simulink model "CL_Xpro_model"  (Simulink 9.1)
settings: Solver=ode45  StartTime=0.0  StopTime=total_time  RelTol=1e-3  EnableMultiTasking=on
values from neighbouring files (symbols this model uses):
  a1 = 16.235    [LoadQuadrotorConst_XPro1a.m]
  a2 = 17.912    [LoadQuadrotorConst_XPro1a.m]
  a3 = 17.914    [LoadQuadrotorConst_XPro1a.m]
  a4 = 18.161    [LoadQuadrotorConst_XPro1a.m]
  b1 = -0.5036    [LoadQuadrotorConst_XPro1a.m]
  b2 = -12.728    [LoadQuadrotorConst_XPro1a.m]
  b3 = -6.5646    [LoadQuadrotorConst_XPro1a.m]
  b4 = -7.4637    [LoadQuadrotorConst_XPro1a.m]
  c = 0.0002    [LoadQuadrotorConst_XPro1a.m]
  c_mi_x = 170*0    (= 0)    [LoadQuadrotorConst_XPro1a.m]
  c_mi_y = 170*0    (= 0)    [LoadQuadrotorConst_XPro1a.m]
  c_mi_z = 40*0    (= 0)    [LoadQuadrotorConst_XPro1a.m]
  co_x = 1.7*0    (= 0)    [LoadQuadrotorConst_XPro1a.m]
  co_y = 1.7*0    (= 0)    [LoadQuadrotorConst_XPro1a.m]
  co_z = 90.7*0    (= 0)    [LoadQuadrotorConst_XPro1a.m]
  controller = 0    [main_sim.m]
  d = 0.5    [LoadQuadrotorConst_XPro1a.m]
  d_omega_R10 = 9.1275    [initial_conditions.m]
  d_omega_R20 = 8.955    [initial_conditions.m]
  d_omega_R30 = 8.61    [initial_conditions.m]
  d_omega_R40 = 8.543    [initial_conditions.m]
  dfi_0 = -0    (= 0)    [initial_conditions.m]
  dpsi_0 = 0    [initial_conditions.m]
  dtheta_0 = 0    [initial_conditions.m]
  dx_0 = 0    [initial_conditions.m]
  dy_0 = 0    [initial_conditions.m]
  dz_0 = 0    [initial_conditions.m]
  f = 5e-6    (= 5e-06)    [LoadQuadrotorConst_XPro1a.m]
  factor = 0.35    [main_sim.m]
  fi_0 = 0    [initial_conditions.m]
  g = 9.807    [K.mat]    (also in LoadQuadrotorConst_XPro1a.m = 0.0008)
  ga = g    [LoadQuadrotorConst_XPro1a.m]
  Gamma = usample(gamma)    [LoadQuadrotorConst_XPro1a.m]
  h = -0.0282    [LoadQuadrotorConst_XPro1a.m]
  input_disturbance = [2 0.4 0.4 0.05]    [K.mat]
  invJac = inv(Jac)    [LoadQuadrotorConst_XPro1a.m]
  Ixx = usample(Ix)    [LoadQuadrotorConst_XPro1a.m]
  Iyy = usample(Iy)    [LoadQuadrotorConst_XPro1a.m]
  Izz = usample(Iz)    [LoadQuadrotorConst_XPro1a.m]
  Jr = 4.86851*0.1    (= 0.486851)    [LoadQuadrotorConst_XPro1a.m]
  L = usample(lx)    [LoadQuadrotorConst_XPro1a.m]
  m = m_nom    [LoadQuadrotorConst_XPro1a.m]
  psi_0 = 0    [initial_conditions.m]
  sensor_noise_weights = [0.1 0.1 0.1 0.01 0.01 0.01 0.0873 0.0873 0.0873 0.00873 0.00873 0.00873]    [K.mat]
  Tau = usample(tau)    [LoadQuadrotorConst_XPro1a.m]
  theta_0 = 0    [initial_conditions.m]
  u_op = [20.5947 0 0 0]    [K.mat]
  V1_WP = 9.1275    [initial_conditions.m]
  V2_WP = 8.955    [initial_conditions.m]
  V3_WP = 8.61    [initial_conditions.m]
  V4_WP = 8.543    [initial_conditions.m]
  x_0 = 0    [initial_conditions.m]
  x_des = [1; 1; 1; 0; 0; 0; 0; 0; pi/12; 0; 0; 0]    [main_sim.m]
  y_0 = 0    [initial_conditions.m]
  z_0 = 0    [initial_conditions.m]
undefined symbols (not defined in the file or in its folder): k, K_lqr
settings Model: SuppressorTable=22 serialization::archive 11 0 6 0 0 0 0 0  Creator=Jake  LastModifiedBy=michaelwang
settings DataIOCC: LimitDataPoints=on  SignalLoggingSaveFormat=ModelDataLogs
settings OptimizationCC: InitFltsAndDblsToZero=on
settings DebuggingCC: SaveWithParameterizedLinksMsg=none  SignalResolutionControl=TryResolveAllWithWarning  SolverPrmCheckMsg=warning  MultiTaskDSMMsg=warning  MultiTaskCondExecSysMsg=none  FcnCallInpInsideContextMsg=warning
settings SFSimCC: SimParseCustomCode=off
settings GRTTargetCC: TargetFcnLib=ansi_tfl_tmw.mat

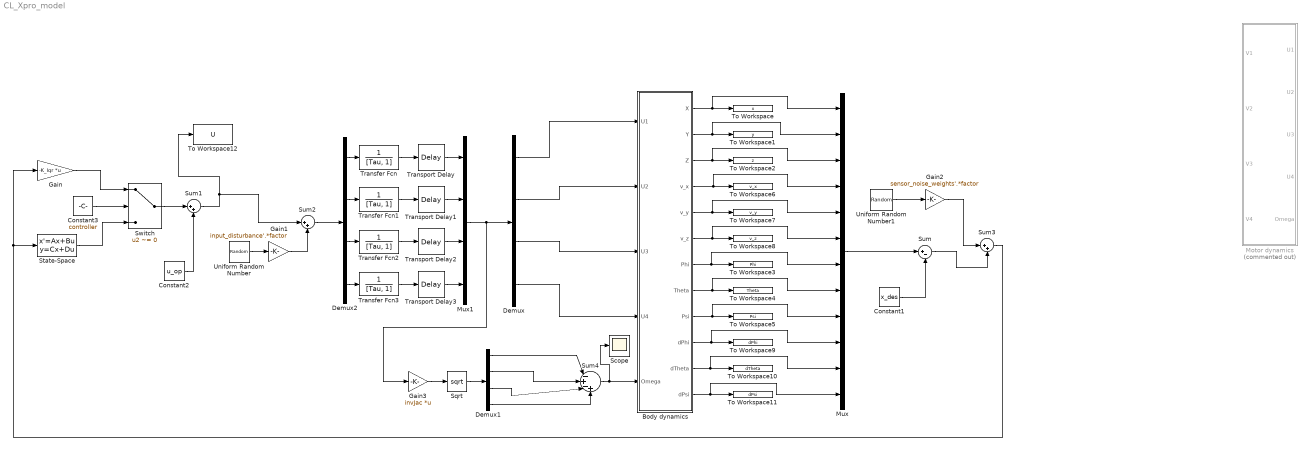
== system CL_Xpro_model ==
  Body dynamics : Subsystem
  Constant1 : Constant  Value=x_des
  Constant2 : Constant  Value=u_op
  Constant3 : Constant  Value=controller
  Demux : Demux
  Demux1 : Demux
  Demux2 : Demux
  Gain : Gain  Gain=-K_lqr  Multiplication=Matrix(K*u)
  Gain1 : Gain  Gain=input_disturbance'.*factor
  Gain2 : Gain  Gain=sensor_noise_weights'.*factor
  Gain3 : Gain  Gain=invJac  Multiplication=Matrix(K*u)
  Motor dynamics : Subsystem  Commented=on
  Mux : Mux  Inputs=12
  Mux1 : Mux
  Scope : Scope
  Sqrt : Sqrt  SaturateOnIntegerOverflow=on
  State-Space : StateSpace  A=k.A  B=k.B  C=k.C  D=k.D  InitialCondition=0
  Sum : Sum  Inputs=|+-
  Sum1 : Sum  Inputs=|++
  Sum2 : Sum  Inputs=|++
  Sum3 : Sum  Inputs=|++
  Sum4 : Sum  Inputs=|-+-+
  Switch : Switch  Criteria=u2 ~= 0
  To Workspace : ToWorkspace  VariableName=x  SaveFormat=Timeseries  SampleTime=-1
  To Workspace1 : ToWorkspace  VariableName=y  SaveFormat=Timeseries  SampleTime=-1
  To Workspace10 : ToWorkspace  VariableName=dTheta  SaveFormat=Timeseries  SampleTime=-1
  To Workspace11 : ToWorkspace  VariableName=dPsi  SaveFormat=Timeseries  SampleTime=-1
  To Workspace12 : ToWorkspace  VariableName=U  SaveFormat=Timeseries  SampleTime=-1
  To Workspace2 : ToWorkspace  VariableName=z  SaveFormat=Timeseries  SampleTime=-1
  To Workspace3 : ToWorkspace  VariableName=Phi  SaveFormat=Timeseries  SampleTime=-1
  To Workspace4 : ToWorkspace  VariableName=Theta  SaveFormat=Timeseries  SampleTime=-1
  To Workspace5 : ToWorkspace  VariableName=Psi  SaveFormat=Timeseries  SampleTime=-1
  To Workspace6 : ToWorkspace  VariableName=v_x  SaveFormat=Timeseries  SampleTime=-1
  To Workspace7 : ToWorkspace  VariableName=v_y  SaveFormat=Timeseries  SampleTime=-1
  To Workspace8 : ToWorkspace  VariableName=v_z  SaveFormat=Timeseries  SampleTime=-1
  To Workspace9 : ToWorkspace  VariableName=dPhi  SaveFormat=Timeseries  SampleTime=-1
  Transfer Fcn{,1..3} (4 alike) : TransferFcn  Denominator=[Tau, 1]
  Transport Delay{,1..3} (4 alike) : TransportDelay  DelayTime=Gamma
  Uniform Random Number : UniformRandomNumber  Minimum=ones(length(input_disturbance),1).*-1  Maximum=ones(length(input_disturbance), 1)  Seed=abs(round(rand().*10))  SampleTime=0.1
  Uniform Random Number1 : UniformRandomNumber  Minimum=ones(length(sensor_noise_weights),1).*-1  Maximum=ones(length(sensor_noise_weights), 1)  Seed=abs(round(rand().*10))  SampleTime=0.1
  wires:
  Body dynamics/1(X) -> Mux/1, To Workspace/1
  Body dynamics/3(Z) -> Mux/3, To Workspace2/1
  Body dynamics/2(Y) -> Mux/2, To Workspace1/1
  Demux/1 -> Body dynamics/1(U1)
  Demux/2 -> Body dynamics/2(U2)
  Demux/3 -> Body dynamics/3(U3)
  Demux/4 -> Body dynamics/4(U4)
  Body dynamics/12(dPsi) -> Mux/12, To Workspace11/1
  Body dynamics/11(dTheta) -> Mux/11, To Workspace10/1
  Body dynamics/10(dPhi) -> Mux/10, To Workspace9/1
  Body dynamics/7(Phi) -> Mux/7, To Workspace3/1
  Body dynamics/8(Theta) -> Mux/8, To Workspace4/1
  Body dynamics/9(Psi) -> Mux/9, To Workspace5/1
  Body dynamics/4(v_x) -> Mux/4, To Workspace6/1
  Body dynamics/5(v_y) -> Mux/5, To Workspace7/1
  Body dynamics/6(v_z) -> Mux/6, To Workspace8/1
  Mux/1 -> Sum/1
  Constant1/1 -> Sum/2
  Sum1/1 -> Sum2/1, To Workspace12/1
  Constant2/1 -> Sum1/2
  Constant3/1 -> Switch/2
  Switch/1 -> Sum1/1
  State-Space/1 -> Switch/3
  Gain/1 -> Switch/1
  Uniform Random Number/1 -> Gain1/1
  Gain1/1 -> Sum2/2
  Uniform Random Number1/1 -> Gain2/1
  Gain2/1 -> Sum3/1
  Sum3/1 -> State-Space/1, Gain/1
  Sum/1 -> Sum3/2
  Gain3/1 -> Sqrt/1
  Sqrt/1 -> Demux1/1
  Sum4/1 -> Scope/1, Body dynamics/5(Omega)
  Demux1/1 -> Sum4/1
  Demux1/2 -> Sum4/2
  Demux1/4 -> Sum4/4
  Demux1/3 -> Sum4/3
  Transfer Fcn/1 -> Transport Delay/1
  Sum2/1 -> Demux2/1
  Demux2/1 -> Transfer Fcn/1
  Transfer Fcn1/1 -> Transport Delay1/1
  Transfer Fcn2/1 -> Transport Delay2/1
  Transfer Fcn3/1 -> Transport Delay3/1
  Demux2/4 -> Transfer Fcn3/1
  Demux2/3 -> Transfer Fcn2/1
  Demux2/2 -> Transfer Fcn1/1
  Transport Delay/1 -> Mux1/1
  Transport Delay1/1 -> Mux1/2
  Transport Delay2/1 -> Mux1/3
  Transport Delay3/1 -> Mux1/4
  Mux1/1 -> Gain3/1, Demux/1

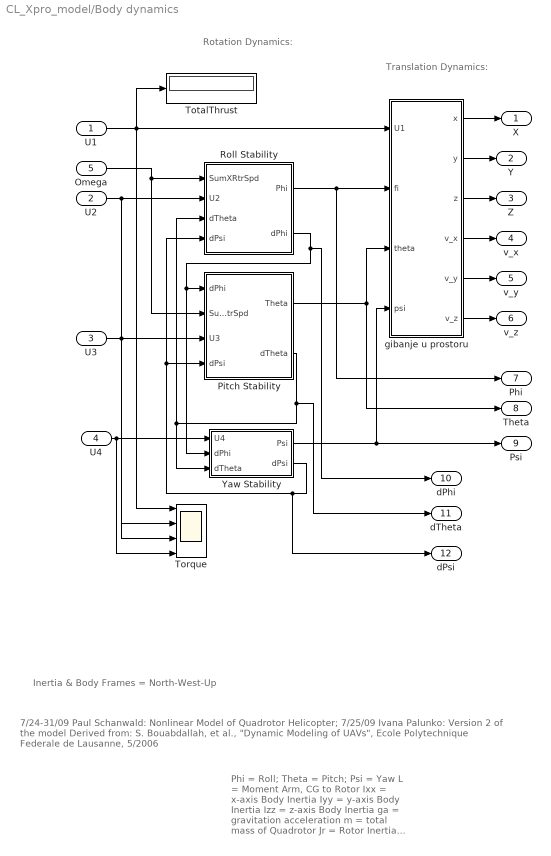
== system CL_Xpro_model/Body dynamics ==
  note: Inertia & Body Frames = North-West-Up
  note: Rotation
      | Dynamics:
  note: Translation
      | Dynamics:
  note: Phi = Roll; Theta = Pitch; Psi = Yaw
      | L = Moment Arm, CG to Rotor
      | Ixx = x-axis Body Inertia
      | Iyy = y-axis Body Inertia
      | Izz = z-axis Body Inertia
      | ga = gravitation acceleration
      | m = total mass of Quadrotor
      | Jr = Rotor Inertia
      | a,b = Volts-to-Rotor Speed Consts
      | c,d,e = RtrSpd-to-Thrust Fcn Consts
      | f,g,h = RtrSpd-to-Drag Fcn Consts
      | Tau = Motor Time Const
  note: 7/24-31/09  Paul Schanwald:  Nonlinear Model of Quadrotor Helicopter; 7/25/09 Ivana Palunko: Version 2 of the model
      | Derived from: S. Bouabdallah, et al., "Dynamic Modeling of UAVs", Ecole Polytechnique Federale de Lausanne, 5/2006
  U1 : Inport
  U2 : Inport  Port=2
  U3 : Inport  Port=3
  U4 : Inport  Port=4
  Omega : Inport  Port=5
  Pitch Stability : Subsystem
  Roll Stability : Subsystem
  Torque : Scope  NumInputPorts=4
  TotalThrust : Display
  Yaw Stability : Subsystem
  gibanje u prostoru : Subsystem
  X : Outport
  Y : Outport  Port=2
  Z : Outport  Port=3
  v_x : Outport  Port=4
  v_y : Outport  Port=5
  v_z : Outport  Port=6
  Phi : Outport  Port=7
  Theta : Outport  Port=8
  Psi : Outport  Port=9
  dPhi : Outport  Port=10
  dTheta : Outport  Port=11
  dPsi : Outport  Port=12
  wires:
  U4/1 -> Yaw Stability/1(U4), Torque/4
  U3/1 -> Pitch Stability/3(U3), Torque/3
  U1/1 -> TotalThrust/1, gibanje u prostoru/1(U1), Torque/1
  gibanje u prostoru/3(z) -> Z/1
  gibanje u prostoru/2(y) -> Y/1
  gibanje u prostoru/1(x) -> X/1
  U2/1 -> Roll Stability/2(U2), Torque/2
  Omega/1 -> Roll Stability/1(SumXRtrSpd), Pitch Stability/2(SumYRtrSpd)
  Roll Stability/2(dPhi) -> dPhi/1, Pitch Stability/1(dPhi), Yaw Stability/2(dPhi)
  Pitch Stability/2(dTheta) -> dTheta/1, Yaw Stability/3(dTheta), Roll Stability/3(dTheta)
  Yaw Stability/2(dPsi) -> dPsi/1, Roll Stability/4(dPsi), Pitch Stability/4(dPsi)
  Roll Stability/1(Phi) -> gibanje u prostoru/2(fi), Phi/1
  Pitch Stability/1(Theta) -> gibanje u prostoru/3(theta), Theta/1
  Yaw Stability/1(Psi) -> Psi/1, gibanje u prostoru/4(psi)
  gibanje u prostoru/6(v_z) -> v_z/1
  gibanje u prostoru/4(v_x) -> v_x/1
  gibanje u prostoru/5(v_y) -> v_y/1

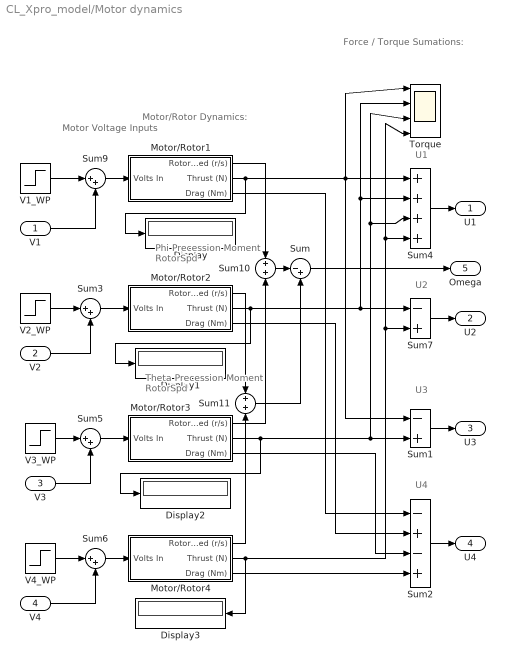
== system CL_Xpro_model/Motor dynamics ==
  note: Theta Precession
      | Moment RotorSpd
  note: Phi Precession
      | Moment RotorSpd
  note: Motor/Rotor
      | Dynamics:
  note: Force / Torque
      | Sumations:
  note: Motor
      | Voltage
      | Inputs
  note: U4
  note: U3
  note: U2
  note: U1
  V1 : Inport
  V2 : Inport  Port=2
  V3 : Inport  Port=3
  V4 : Inport  Port=4
  Display{,1..3} (4 alike) : Display
  Motor/Rotor1 : Subsystem
  Motor/Rotor2 : Subsystem
  Motor/Rotor3 : Subsystem
  Motor/Rotor4 : Subsystem
  Sum : Sum  Inputs=|-+
  Sum1 : Sum  Inputs=-+
  Sum10 : Sum  Inputs=+|+
  Sum11 : Sum  Inputs=+|+
  Sum2 : Sum  Inputs=-+-+
  Sum{3,5..6,9} (4 alike) : Sum  Inputs=|++
  Sum4 : Sum  Inputs=++++
  Sum7 : Sum  Inputs=-+
  Torque : Scope  NumInputPorts=4
  V1_WP : Step  Time=0  Before=V1_WP  After=V1_WP  SampleTime=0
  V2_WP : Step  Time=0  Before=V2_WP  After=V2_WP  SampleTime=0
  V3_WP : Step  Time=0  Before=V3_WP  After=V3_WP  SampleTime=0
  V4_WP : Step  Time=0  Before=V4_WP  After=V4_WP  SampleTime=0
  U1 : Outport
  U2 : Outport  Port=2
  U3 : Outport  Port=3
  U4 : Outport  Port=4
  Omega : Outport  Port=5
  wires:
  Sum11/1 -> Sum/2
  Sum10/1 -> Sum/1
  Motor/Rotor4/1(Rotor Speed (r/s)) -> Sum11/2
  Motor/Rotor4/2(Thrust (N)) -> Display3/1, Torque/4, Sum4/4, Sum7/2
  Motor/Rotor4/3(Drag (Nm)) -> Sum2/4
  Motor/Rotor3/3(Drag (Nm)) -> Sum2/3
  Motor/Rotor3/1(Rotor Speed (r/s)) -> Sum10/2
  Motor/Rotor3/2(Thrust (N)) -> Display2/1, Torque/3, Sum4/3, Sum1/2
  Motor/Rotor2/1(Rotor Speed (r/s)) -> Sum11/1
  Motor/Rotor2/3(Drag (Nm)) -> Sum2/2
  Motor/Rotor2/2(Thrust (N)) -> Display1/1, Torque/2, Sum4/2, Sum7/1
  Motor/Rotor1/1(Rotor Speed (r/s)) -> Sum10/1
  Motor/Rotor1/3(Drag (Nm)) -> Sum2/1
  Motor/Rotor1/2(Thrust (N)) -> Display/1, Sum4/1, Torque/1, Sum1/1
  Sum4/1 -> U1/1
  Sum/1 -> Omega/1
  Sum7/1 -> U2/1
  Sum1/1 -> U3/1
  Sum2/1 -> U4/1
  Sum9/1 -> Motor/Rotor1/1(Volts In)
  V1_WP/1 -> Sum9/1
  V2_WP/1 -> Sum3/1
  Sum3/1 -> Motor/Rotor2/1(Volts In)
  V3_WP/1 -> Sum5/1
  Sum5/1 -> Motor/Rotor3/1(Volts In)
  V4_WP/1 -> Sum6/1
  Sum6/1 -> Motor/Rotor4/1(Volts In)
  V1/1 -> Sum9/2
  V2/1 -> Sum3/2
  V3/1 -> Sum5/2
  V4/1 -> Sum6/2

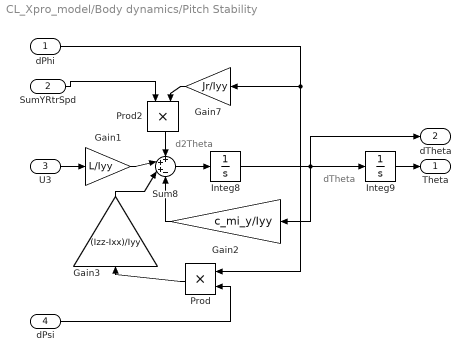
== system CL_Xpro_model/Body dynamics/Pitch Stability ==
  note: d2Theta
  note: dTheta
  dPhi : Inport
  SumYRtrSpd : Inport  Port=2
  U3 : Inport  Port=3
  dPsi : Inport  Port=4
  Gain1 : Gain  Gain=L/Iyy
  Gain2 : Gain  Gain=c_mi_y/Iyy
  Gain3 : Gain  Gain=(Izz-Ixx)/Iyy
  Gain7 : Gain  Gain=Jr/Iyy
  Integ8 : Integrator  InitialCondition=dtheta_0
  Integ9 : Integrator  InitialCondition=theta_0  UpperSaturationLimit=pi/2  LowerSaturationLimit=-pi/2
  Prod : Product  RndMeth=Zero
  Prod2 : Product  RndMeth=Zero
  Sum8 : Sum  Inputs=+++-
  Theta : Outport
  dTheta : Outport  Port=2
  wires:
  Gain2/1 -> Sum8/4
  dPhi/1 -> Prod/1, Gain7/1
  Integ9/1 -> Theta/1
  U3/1 -> Gain1/1
  SumYRtrSpd/1 -> Prod2/1
  dPsi/1 -> Prod/2
  Integ8/1 -> dTheta/1, Integ9/1, Gain2/1
  Sum8/1 -> Integ8/1
  Gain1/1 -> Sum8/2
  Gain7/1 -> Prod2/2
  Gain3/1 -> Sum8/3
  Prod/1 -> Gain3/1
  Prod2/1 -> Sum8/1

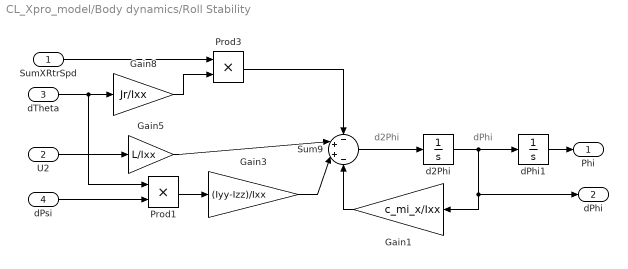
== system CL_Xpro_model/Body dynamics/Roll Stability ==
  note: d2Phi
  note: dPhi
  SumXRtrSpd : Inport
  U2 : Inport  Port=2
  dTheta : Inport  Port=3
  dPsi : Inport  Port=4
  Gain1 : Gain  Gain=c_mi_x/Ixx
  Gain3 : Gain  Gain=(Iyy-Izz)/Ixx
  Gain5 : Gain  Gain=L/Ixx
  Gain8 : Gain  Gain=Jr/Ixx
  Prod1 : Product  RndMeth=Zero
  Prod3 : Product  RndMeth=Zero
  Sum9 : Sum  Inputs=-++-
  d2Phi : Integrator  InitialCondition=dfi_0
  dPhi1 : Integrator  InitialCondition=fi_0  UpperSaturationLimit=pi/2  LowerSaturationLimit=-pi/2
  Phi : Outport
  dPhi : Outport  Port=2
  wires:
  dPsi/1 -> Prod1/2
  dTheta/1 -> Prod1/1, Gain8/1
  Prod3/1 -> Sum9/1
  SumXRtrSpd/1 -> Prod3/1
  Gain8/1 -> Prod3/2
  dPhi1/1 -> Phi/1
  U2/1 -> Gain5/1
  d2Phi/1 -> Gain1/1, dPhi/1, dPhi1/1
  Sum9/1 -> d2Phi/1
  Gain5/1 -> Sum9/2
  Gain1/1 -> Sum9/4
  Gain3/1 -> Sum9/3
  Prod1/1 -> Gain3/1

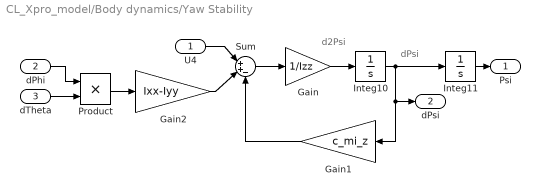
== system CL_Xpro_model/Body dynamics/Yaw Stability ==
  note: dPsi
  note: d2Psi
  U4 : Inport
  dPhi : Inport  Port=2
  dTheta : Inport  Port=3
  Gain : Gain  Gain=1/Izz
  Gain1 : Gain  Gain=c_mi_z
  Gain2 : Gain  Gain=Ixx-Iyy
  Integ10 : Integrator  InitialCondition=dpsi_0
  Integ11 : Integrator  InitialCondition=psi_0
  Product : Product  RndMeth=Zero
  Sum : Sum  Inputs=|++-
  Psi : Outport
  dPsi : Outport  Port=2
  wires:
  Sum/1 -> Gain/1
  U4/1 -> Sum/1
  Integ11/1 -> Psi/1
  Gain/1 -> Integ10/1
  Integ10/1 -> Gain1/1, dPsi/1, Integ11/1
  Gain1/1 -> Sum/3
  Gain2/1 -> Sum/2
  dPhi/1 -> Product/1
  dTheta/1 -> Product/2
  Product/1 -> Gain2/1

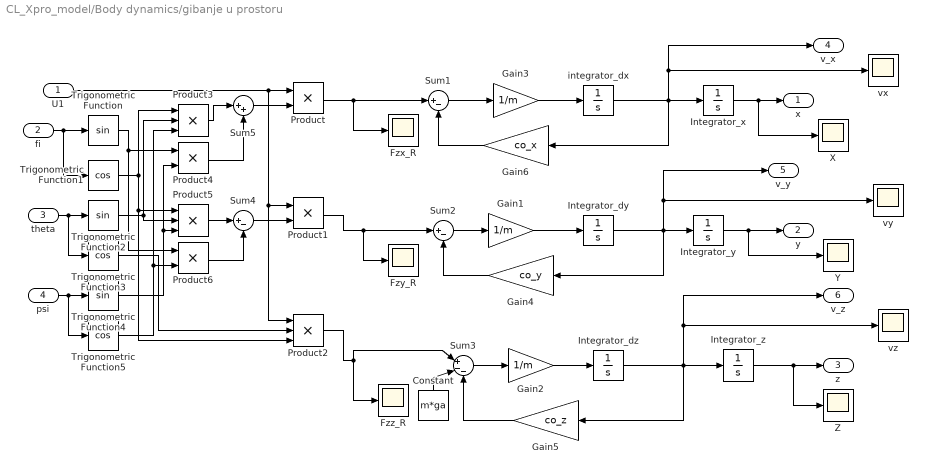
== system CL_Xpro_model/Body dynamics/gibanje u prostoru ==
  U1 : Inport
  fi : Inport  Port=2
  theta : Inport  Port=3
  psi : Inport  Port=4
  Constant : Constant  Value=m*ga
  Fzx_R : Scope
  Fzy_R : Scope
  Fzz_R : Scope
  Gain1 : Gain  Gain=1/m
  Gain2 : Gain  Gain=1/m
  Gain3 : Gain  Gain=1/m
  Gain4 : Gain  Gain=co_y
  Gain5 : Gain  Gain=co_z
  Gain6 : Gain  Gain=co_x
  Integrator_dy : Integrator  InitialCondition=dy_0  LimitOutput=on  UpperSaturationLimit=10  LowerSaturationLimit=-10
  Integrator_dz : Integrator  InitialCondition=dz_0  LimitOutput=on  UpperSaturationLimit=10  LowerSaturationLimit=-10
  Integrator_x : Integrator  InitialCondition=x_0
  Integrator_y : Integrator  InitialCondition=y_0
  Integrator_z : Integrator  InitialCondition=z_0
  Product{,1,4,6} (4 alike) : Product  RndMeth=Zero
  Product2 : Product  Inputs=3  RndMeth=Zero
  Product3 : Product  Inputs=3  RndMeth=Zero
  Product5 : Product  Inputs=3  RndMeth=Zero
  Sum1 : Sum  Inputs=|+-
  Sum2 : Sum  Inputs=|+-
  Sum3 : Sum  Inputs=|+--
  Sum4 : Sum  Inputs=|+-
  Sum5 : Sum  Inputs=|++
  Trigonometric Function : Trigonometry
  Trigonometric Function1 : Trigonometry  Operator=cos
  Trigonometric Function2 : Trigonometry
  Trigonometric Function3 : Trigonometry  Operator=cos
  Trigonometric Function4 : Trigonometry
  Trigonometric Function5 : Trigonometry  Operator=cos
  X : Scope
  Y : Scope
  Z : Scope
  integrator_dx : Integrator  InitialCondition=dx_0  LimitOutput=on  UpperSaturationLimit=10  LowerSaturationLimit=-10
  vx : Scope
  vy : Scope
  vz : Scope
  x : Outport
  y : Outport  Port=2
  z : Outport  Port=3
  v_x : Outport  Port=4
  v_y : Outport  Port=5
  v_z : Outport  Port=6
  wires:
  Gain5/1 -> Sum3/3
  Constant/1 -> Sum3/2
  Gain4/1 -> Sum2/2
  Sum3/1 -> Gain2/1
  Gain6/1 -> Sum1/2
  Product2/1 -> Sum3/1, Fzz_R/1
  Sum2/1 -> Gain1/1
  Product1/1 -> Fzy_R/1, Sum2/1
  Gain2/1 -> Integrator_dz/1
  Sum1/1 -> Gain3/1
  Product/1 -> Fzx_R/1, Sum1/1
  U1/1 -> Product/1, Product1/1, Product2/1
  Integrator_y/1 -> Y/1, y/1
  Integrator_x/1 -> X/1, x/1
  Integrator_z/1 -> Z/1, z/1
  integrator_dx/1 -> Gain6/1, vx/1, v_x/1, Integrator_x/1
  Integrator_dy/1 -> Gain4/1, Integrator_y/1, vy/1, v_y/1
  Integrator_dz/1 -> vz/1, v_z/1, Gain5/1, Integrator_z/1
  Gain1/1 -> Integrator_dy/1
  Gain3/1 -> integrator_dx/1
  Sum4/1 -> Product1/2
  Sum5/1 -> Product/2
  Product3/1 -> Sum5/1
  Product4/1 -> Sum5/2
  Product5/1 -> Sum4/1
  Product6/1 -> Sum4/2
  psi/1 -> Trigonometric Function4/1, Trigonometric Function5/1
  theta/1 -> Trigonometric Function2/1, Trigonometric Function3/1
  fi/1 -> Trigonometric Function/1, Trigonometric Function1/1
  Trigonometric Function/1 -> Product4/1, Product6/1
  Trigonometric Function1/1 -> Product3/1, Product5/1, Product2/3
  Trigonometric Function2/1 -> Product3/2, Product5/2
  Trigonometric Function5/1 -> Product3/3, Product6/2
  Trigonometric Function4/1 -> Product4/2, Product5/3
  Trigonometric Function3/1 -> Product2/2

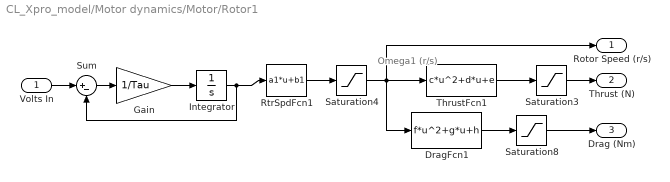
== system CL_Xpro_model/Motor dynamics/Motor/Rotor1 ==
  note: Omega1
      | (r/s)
  Volts In : Inport
  DragFcn1 : Fcn  Expr=f*u^2+g*u+h
  Gain : Gain  Gain=1/Tau
  Integrator : Integrator  InitialCondition=d_omega_R10
  RtrSpdFcn1 : Fcn  Expr=a1*u+b1
  Saturation3 : Saturate  UpperLimit=15  LowerLimit=0
  Saturation4 : Saturate  UpperLimit=250  LowerLimit=0
  Saturation8 : Saturate  UpperLimit=1  LowerLimit=0
  Sum : Sum  Inputs=|+-
  ThrustFcn1 : Fcn  Expr=c*u^2+d*u+e
  Rotor Speed (r/s) : Outport
  Thrust (N) : Outport  Port=2
  Drag (Nm) : Outport  Port=3
  wires:
  Volts In/1 -> Sum/1
  Sum/1 -> Gain/1
  Integrator/1 -> RtrSpdFcn1/1, Sum/2
  Gain/1 -> Integrator/1
  Saturation3/1 -> Thrust (N)/1
  Saturation8/1 -> Drag (Nm)/1
  DragFcn1/1 -> Saturation8/1
  Saturation4/1 -> Rotor Speed (r/s)/1, DragFcn1/1, ThrustFcn1/1
  RtrSpdFcn1/1 -> Saturation4/1
  ThrustFcn1/1 -> Saturation3/1

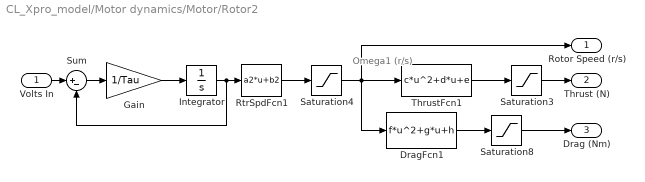
== system CL_Xpro_model/Motor dynamics/Motor/Rotor2 ==
  note: Omega1
      | (r/s)
  Volts In : Inport
  DragFcn1 : Fcn  Expr=f*u^2+g*u+h
  Gain : Gain  Gain=1/Tau
  Integrator : Integrator  InitialCondition=d_omega_R20
  RtrSpdFcn1 : Fcn  Expr=a2*u+b2
  Saturation3 : Saturate  UpperLimit=15  LowerLimit=0
  Saturation4 : Saturate  UpperLimit=250  LowerLimit=0
  Saturation8 : Saturate  UpperLimit=1  LowerLimit=0
  Sum : Sum  Inputs=|+-
  ThrustFcn1 : Fcn  Expr=c*u^2+d*u+e
  Rotor Speed (r/s) : Outport
  Thrust (N) : Outport  Port=2
  Drag (Nm) : Outport  Port=3
  wires:
  Volts In/1 -> Sum/1
  Sum/1 -> Gain/1
  Integrator/1 -> RtrSpdFcn1/1, Sum/2
  Gain/1 -> Integrator/1
  Saturation3/1 -> Thrust (N)/1
  Saturation8/1 -> Drag (Nm)/1
  DragFcn1/1 -> Saturation8/1
  ThrustFcn1/1 -> Saturation3/1
  Saturation4/1 -> Rotor Speed (r/s)/1, DragFcn1/1, ThrustFcn1/1
  RtrSpdFcn1/1 -> Saturation4/1

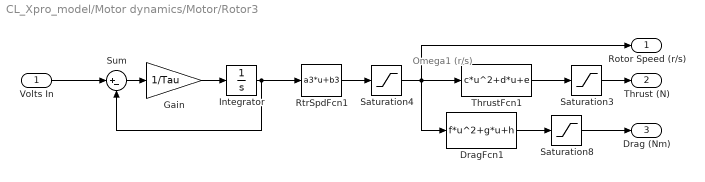
== system CL_Xpro_model/Motor dynamics/Motor/Rotor3 ==
  note: Omega1
      | (r/s)
  Volts In : Inport
  DragFcn1 : Fcn  Expr=f*u^2+g*u+h
  Gain : Gain  Gain=1/Tau
  Integrator : Integrator  InitialCondition=d_omega_R30
  RtrSpdFcn1 : Fcn  Expr=a3*u+b3
  Saturation3 : Saturate  UpperLimit=15  LowerLimit=0
  Saturation4 : Saturate  UpperLimit=250  LowerLimit=0
  Saturation8 : Saturate  UpperLimit=1  LowerLimit=0
  Sum : Sum  Inputs=|+-
  ThrustFcn1 : Fcn  Expr=c*u^2+d*u+e
  Rotor Speed (r/s) : Outport
  Thrust (N) : Outport  Port=2
  Drag (Nm) : Outport  Port=3
  wires:
  Volts In/1 -> Sum/1
  Sum/1 -> Gain/1
  Integrator/1 -> RtrSpdFcn1/1, Sum/2
  Gain/1 -> Integrator/1
  Saturation3/1 -> Thrust (N)/1
  Saturation8/1 -> Drag (Nm)/1
  DragFcn1/1 -> Saturation8/1
  ThrustFcn1/1 -> Saturation3/1
  Saturation4/1 -> Rotor Speed (r/s)/1, DragFcn1/1, ThrustFcn1/1
  RtrSpdFcn1/1 -> Saturation4/1

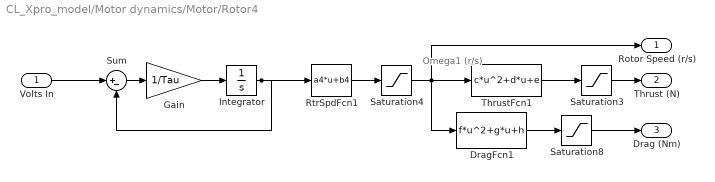
== system CL_Xpro_model/Motor dynamics/Motor/Rotor4 ==
  note: Omega1
      | (r/s)
  Volts In : Inport
  DragFcn1 : Fcn  Expr=f*u^2+g*u+h
  Gain : Gain  Gain=1/Tau
  Integrator : Integrator  InitialCondition=d_omega_R40
  RtrSpdFcn1 : Fcn  Expr=a4*u+b4
  Saturation3 : Saturate  UpperLimit=15  LowerLimit=0
  Saturation4 : Saturate  UpperLimit=250  LowerLimit=0
  Saturation8 : Saturate  UpperLimit=1  LowerLimit=0
  Sum : Sum  Inputs=|+-
  ThrustFcn1 : Fcn  Expr=c*u^2+d*u+e
  Rotor Speed (r/s) : Outport
  Thrust (N) : Outport  Port=2
  Drag (Nm) : Outport  Port=3
  wires:
  Volts In/1 -> Sum/1
  Sum/1 -> Gain/1
  Integrator/1 -> RtrSpdFcn1/1, Sum/2
  Gain/1 -> Integrator/1
  Saturation3/1 -> Thrust (N)/1
  Saturation8/1 -> Drag (Nm)/1
  DragFcn1/1 -> Saturation8/1
  ThrustFcn1/1 -> Saturation3/1
  Saturation4/1 -> Rotor Speed (r/s)/1, DragFcn1/1, ThrustFcn1/1
  RtrSpdFcn1/1 -> Saturation4/1
